simulink model "SoC"  (R2023b)
settings: Solver=FixedStepAuto  StartTime=0.0  StopTime=14000  RelTol=1e-3
libraries: BatteryEstimators x4
settings Model: Creator=dwegg  LastModifiedBy=joser
settings SolverCC: AlgebraicLoopSolver=TrustRegion
settings OptimizationCC: DefaultParameterBehavior=Inlined
settings DebuggingCC: UnconnectedInputMsg=warning  UnconnectedOutputMsg=warning  UnconnectedLineMsg=warning  ArithmeticOperatorsInVariantConditions=warning
settings ModelReferenceCC: EnableRefExpFcnMdlSchedulingChecks=on
settings SFSimCC: CustomCodeUndefinedFunction=UseInterfaceOnly
settings RTWCC: Description=INTECRIO Real-Time Target  SystemTargetFile=irt.tlc  TemplateMakefile=irt_default_tmf
settings STFCustomTargetCC: UtilityFuncGeneration=Shared location  MatFileLogging=on  GRTInterface=on  SystemTargetFile=irt.tlc
settings GRTTargetCC: UtilityFuncGeneration=Shared location  ParMdlRefBuildCompliant=off  CompOptLevelCompliant=off  ConcurrentExecutionCompliant=off  CombineOutputUpdateFcns=off  CPPClassGenCompliant=off  GRTInterface=on  UseToolchainInfoCompliant=off  GenerateASAP2=on

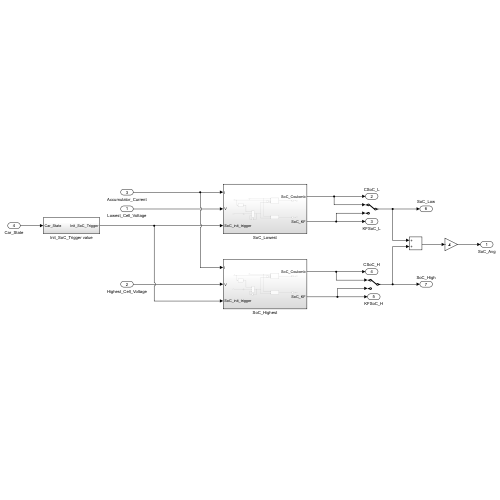
[thumbnail: Simulink's stored preview of the top-level diagram]
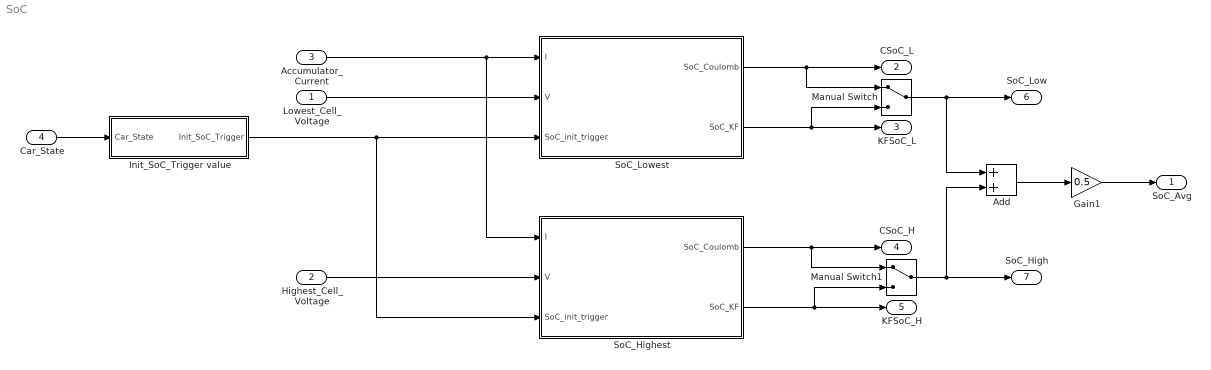
== system SoC ==
  Lowest_Cell_Voltage : Inport
  Highest_Cell_Voltage : Inport  Port=2
  Accumulator_Current : Inport  Port=3
  Car_State : Inport  Port=4
  Add : Sum
  Gain1 : Gain  Gain=0.5
  Init_SoC_Trigger value : Subsystem
  Manual Switch : ManualSwitch
  Manual Switch1 : ManualSwitch
  SoC_Highest : Subsystem
  SoC_Lowest : Subsystem
  SoC_Avg : Outport
  CSoC_L : Outport  Port=2
  KFSoC_L : Outport  Port=3
  CSoC_H : Outport  Port=4
  KFSoC_H : Outport  Port=5
  SoC_Low : Outport  Port=6
  SoC_High : Outport  Port=7
  wires:
  Lowest_Cell_Voltage/1 -> SoC_Lowest/2(V)
  Init_SoC_Trigger value/1(Init_SoC_Trigger) -> SoC_Highest/3(SoC_init_trigger), SoC_Lowest/3(SoC_init_trigger)
  Accumulator_Current/1 -> SoC_Highest/1(I), SoC_Lowest/1(I)
  SoC_Lowest/1(SoC_Coulomb) -> CSoC_L/1, Manual Switch/1
  SoC_Lowest/2(SoC_KF) -> KFSoC_L/1, Manual Switch/2
  SoC_Highest/2(SoC_KF) -> KFSoC_H/1, Manual Switch1/2
  SoC_Highest/1(SoC_Coulomb) -> CSoC_H/1, Manual Switch1/1
  Manual Switch/1 -> SoC_Low/1, Add/1
  Manual Switch1/1 -> SoC_High/1, Add/2
  Add/1 -> Gain1/1
  Gain1/1 -> SoC_Avg/1
  Highest_Cell_Voltage/1 -> SoC_Highest/2(V)
  Car_State/1 -> Init_SoC_Trigger value/1(Car_State)

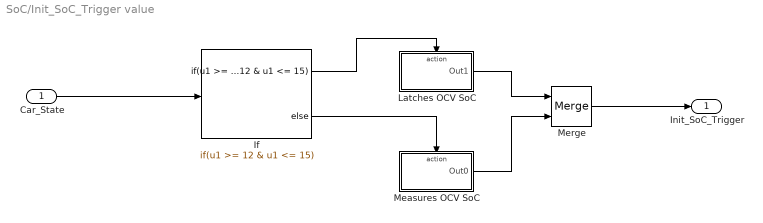
== system SoC/Init_SoC_Trigger value ==
  Car_State : Inport
  If : If  IfExpression=u1 >= 12 & u1 <= 15
  Latches OCV SoC : Subsystem  TreatAsAtomicUnit=on
  Measures OCV SoC : Subsystem  TreatAsAtomicUnit=on
  Merge : Merge
  Init_SoC_Trigger : Outport  VectorParamsAs1DForOutWhenUnconnected=off
  wires:
  Car_State/1 -> If/1
  If/1 -> Latches OCV SoC/Action
  If/2 -> Measures OCV SoC/Action
  Measures OCV SoC/1(Out0) -> Merge/2
  Latches OCV SoC/1(Out1) -> Merge/1
  Merge/1 -> Init_SoC_Trigger/1

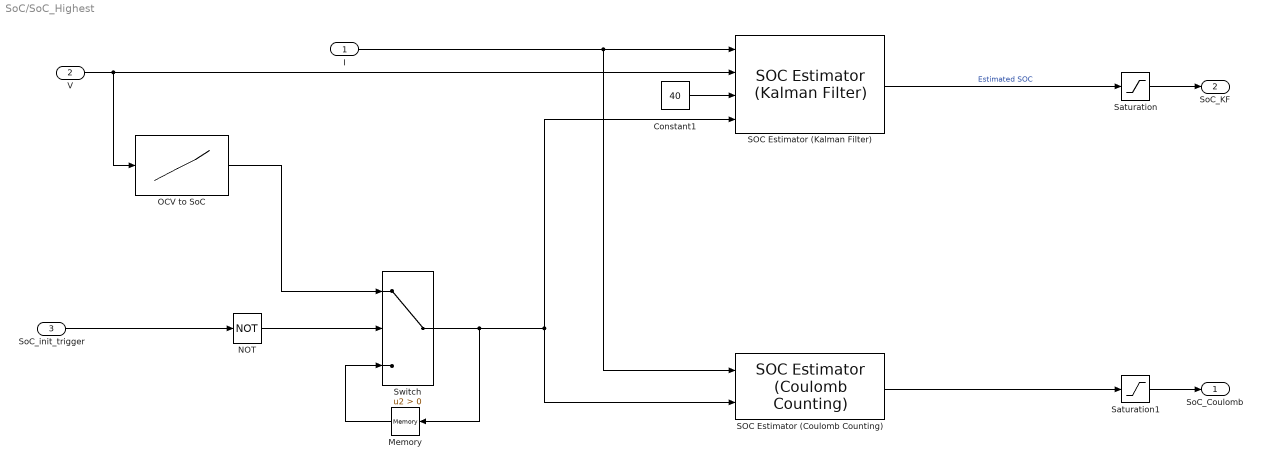
== system SoC/SoC_Highest ==
  I : Inport
  V : Inport  Port=2
  SoC_init_trigger : Inport  Port=3
  Constant1 : Constant  Value=40
  Memory : Memory
  NOT : Logic  Operator=NOT  IconShape=distinctive  AllPortsSameDT=off  OutDataTypeStr=boolean
  OCV to SoC : Lookup_n-D  NumberOfTableDimensions=1  BreakpointsForDimension1=|  Table=|  InternalRulePriority=Speed  RndMeth=Simplest
      BreakpointsForDimension1=|
      | [2.94959022892031
      | 3.21416977318498
      | 3.34338141328538
      | 3.38823547157865
      | 3.42107134634789
      | 3.48650481123582
      | 3.51335866761468
      | 3.54070339538832
      | 3.56968305677313
      | 3.63185877907628
      | 3.63255716896237
      | 3.64803371545993
      | 3.66548496788278
      | 3.66563518858557
      | 3.72681148156897
      | 3.76406010705888
      | 3.77075982343748
      | 3.84270466053206
      | 3.84295206305238
      | 3.90164564850831
      | 3.96498508551296
      | 3.96615700649565
      | 4.04797311953080
      | 4.07602027520885
      | 4.10936207844059
      | 4.18278376875771]
      Table=|
      | [0.00364887820512694
      | 0.0406322115384605
      | 0.0806891025641018
      | 0.120744391025641
      | 0.160802083333333
      | 0.200854967948718
      | 0.240911057692307
      | 0.280964743589743
      | 0.321025641025641
      | 0.361079326923077
      | 0.401137019230769
      | 0.441193910256410
      | 0.481247596153846
      | 0.521301282051282
      | 0.561357371794872
      | 0.601413461538462
      | 0.641456730769231
      | 0.681509615384616
      | 0.721566506410257
      | 0.761620993589744
      | 0.801677884615385
      | 0.841734775641026
      | 0.881788461538462
      | 0.921837339743590
      | 0.961899038461539
      | 0.998685256410256]
  SOC Estimator (Coulomb Counting) : BatteryEstimators/SOC Estimator (Coulomb Counting)  CurrentInputPartition=on  AH=2.6*5  Ts=1
  SOC Estimator (Kalman Filter) : BatteryEstimators/SOC Estimator (Kalman Filter)  CurrentInputPartition=off  filterType=Unscented Kalman filter  alpha=1  beta=2  kappa=0  Q=|  R=1e-3  P0=[1e-8 0; 0 1]  Ts=.025  SOC_vec=|  T_vec=[40+273]  R0_mat=|  R1_mat=|  tau1_mat=|  V0_mat=|  AH=12.5
      Q=|
      | [1e-9 0;
      | 0 1e-9]
      SOC_vec=|
      | [0.00364887820512694
      | 0.0406322115384605
      | 0.0806891025641018
      | 0.120744391025641
      | 0.160802083333333
      | 0.200854967948718
      | 0.240911057692307
      | 0.280964743589743
      | 0.321025641025641
      | 0.361079326923077
      | 0.401137019230769
      | 0.441193910256410
      | 0.481247596153846
      | 0.521301282051282
      | 0.561357371794872
      | 0.601413461538462
      | 0.641456730769231
      | 0.681509615384616
      | 0.721566506410257
      | 0.761620993589744
      | 0.801677884615385
      | 0.841734775641026
      | 0.881788461538462
      | 0.921837339743590
      | 0.961899038461539
      | 0.998685256410256]
      R0_mat=|
      | [0.0100233572019649
      | 0.0262776800968641
      | 0.0363128958641671
      | 0.0100113094505490
      | 0.0286486807277356
      | 0.0149767890889632
      | 0.0144578183036739
      | 0.0281525249750630
      | 0.0100063258437773
      | 0.0279749794813750
      | 0.0217631517067980
      | 0.0101315932150831
      | 0.0204969050806245
      | 0.0100036904397663
      | 0.0234196819492359
      | 0.0285785961250009
      | 0.0100010777636376
      | 0.0285512087508609
      | 0.0138948165245514
      | 0.0152455499563035
      | 0.0271834062533151
      | 0.00999543636151631
      | 0.0233190816650244
      | 0.0174459063712128
      | 0.00997795030699019
      | 0.0103822437854372]
      R1_mat=|
      | [0.000499569519126077
      | 0.000566384348175598
      | 0.000620513515330880
      | 0.000501834816986178
      | 0.000588952675343360
      | 0.000529656285954493
      | 0.000517421423028936
      | 0.000587687483006353
      | 0.000500912051109555
      | 0.000578364620913254
      | 0.000558041081149625
      | 0.000501034112890869
      | 0.000552539389402844
      | 0.000501551598015617
      | 0.000557375879673445
      | 0.000589089399714461
      | 0.000500612734241474
      | 0.000591500744740345
      | 0.000524954003879735
      | 0.000521737226573142
      | 0.000584978563699472
      | 0.000501333485097591
      | 0.000556455598375632
      | 0.000536187820761028
      | 0.000499639620215416
      | 0.000507199196258293]
      tau1_mat=|
      | [9.99999965128907
      | 9.98553115975498
      | 9.98319684629733
      | 9.99994867285566
      | 9.97472406054001
      | 9.99688938669185
      | 9.99522470508715
      | 9.98942560461659
      | 9.99999050049701
      | 9.99099110217109
      | 9.99738841102412
      | 9.99884730510879
      | 9.99441213972015
      | 9.99999487663704
      | 9.99510659168373
      | 9.99771333296480
      | 9.99992313725565
      | 9.99397201956115
      | 10.0015797566463
      | 9.99642521143648
      | 9.99339019420605
      | 9.99998885830201
      | 9.98301776831365
      | 9.99305327108613
      | 9.99970822142190
      | 9.99116677405533]
      V0_mat=|
      | [2.94959022892031
      | 3.21416977318498
      | 3.34338141328538
      | 3.38823547157865
      | 3.50107134634789
      | 3.48650481123582
      | 3.51335866761468
      | 3.58070339538832
      | 3.56968305677313
      | 3.63985877907628
      | 3.63255716896237
      | 3.62803371545993
      | 3.67548496788278
      | 3.66563518858557
      | 3.72681148156897
      | 3.76466010705888
      | 3.76075982343748
      | 3.85370466053206
      | 3.84295206305238
      | 3.90164564850831
      | 3.96498508551296
      | 3.96615700649565
      | 4.04797311953080
      | 4.07602027520885
      | 4.10936207844059
      | 4.18278376875771]
      link override Kalman Filter/EKBF/Jacobian/2-D Lookup Table C1: NumberOfTableDimensions=1
      link override Kalman Filter/EKBF/Jacobian/2-D Lookup Table R0: NumberOfTableDimensions=1
      link override Kalman Filter/EKBF/Jacobian/2-D Lookup Table R1: NumberOfTableDimensions=1
      link override Kalman Filter/EKBF/Jacobian/2-D Lookup Table V0: NumberOfTableDimensions=1
      link override Kalman Filter/EKBF/Jacobian/2-D Lookup Table dV0: NumberOfTableDimensions=1
      link override Kalman Filter/EKF/Jacobian/2-D Lookup Table C1: NumberOfTableDimensions=1
      link override Kalman Filter/EKF/Jacobian/2-D Lookup Table R0: NumberOfTableDimensions=1
      link override Kalman Filter/EKF/Jacobian/2-D Lookup Table R1: NumberOfTableDimensions=1
      link override Kalman Filter/EKF/Jacobian/2-D Lookup Table V0: NumberOfTableDimensions=1
      link override Kalman Filter/EKF/Jacobian/2-D Lookup Table dV0: NumberOfTableDimensions=1
      link override Kalman Filter/UKBF/Prediction-correction/Measurement function/Measurement function/OCV Table: NumberOfTableDimensions=1
      link override Kalman Filter/UKBF/Prediction-correction/Measurement function/Measurement function/R0 Table: NumberOfTableDimensions=1
      link override Kalman Filter/UKBF/Prediction-correction/State function/State function/C1: NumberOfTableDimensions=1
      link override Kalman Filter/UKBF/Prediction-correction/State function/State function/R1: NumberOfTableDimensions=1
      link override Kalman Filter/UKF/Prediction/Measurement function/Measurement function/OCV Table: NumberOfTableDimensions=1
      link override Kalman Filter/UKF/Prediction/Measurement function/Measurement function/R0 Table: NumberOfTableDimensions=1
      link override Kalman Filter/UKF/Prediction/State function/State function/C1: NumberOfTableDimensions=1
      link override Kalman Filter/UKF/Prediction/State function/State function/R1: NumberOfTableDimensions=1
  Saturation : Saturate  UpperLimit=100  LowerLimit=0
  Saturation1 : Saturate  UpperLimit=100  LowerLimit=0
  Switch : Switch  Criteria=u2 > Threshold  ZeroCross=off  SaturateOnIntegerOverflow=off  InputSameDT=off
  SoC_Coulomb : Outport  VectorParamsAs1DForOutWhenUnconnected=off
  SoC_KF : Outport  Port=2
  wires:
  Saturation1/1 -> SoC_Coulomb/1
  Saturation/1 -> SoC_KF/1
  SoC_init_trigger/1 -> NOT/1
  NOT/1 -> Switch/2
  Memory/1 -> Switch/3
  OCV to SoC/1 -> Switch/1
  V/1 -> SOC Estimator (Kalman Filter)/2, OCV to SoC/1
  Switch/1 -> SOC Estimator (Coulomb Counting)/2, SOC Estimator (Kalman Filter)/4, Memory/1
  I/1 -> SOC Estimator (Kalman Filter)/1, SOC Estimator (Coulomb Counting)/1
  Constant1/1 -> SOC Estimator (Kalman Filter)/3
  SOC Estimator (Kalman Filter)/1 -> Saturation/1  "Estimated SOC"
  SOC Estimator (Coulomb Counting)/1 -> Saturation1/1

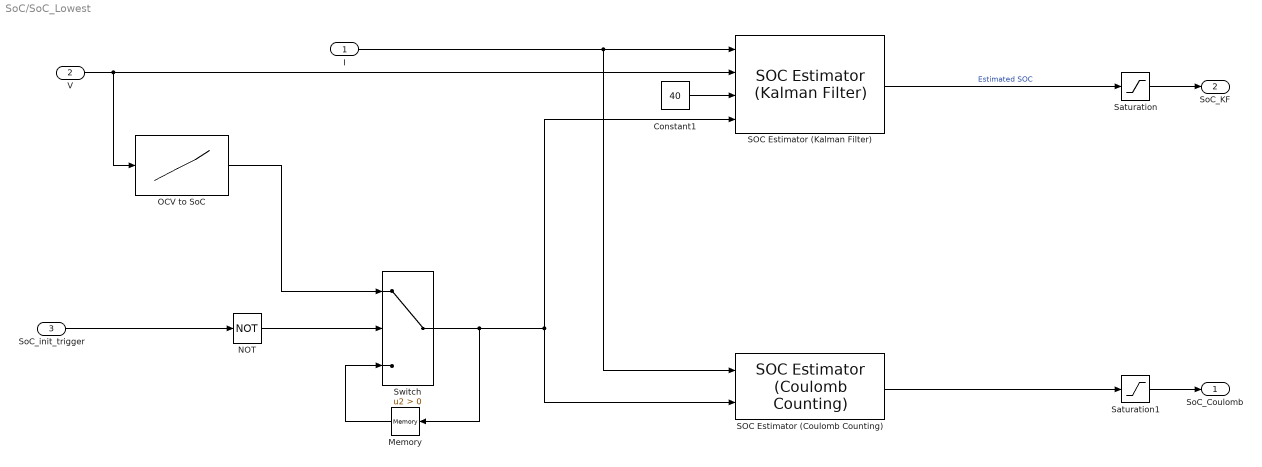
== system SoC/SoC_Lowest ==
  I : Inport
  V : Inport  Port=2
  SoC_init_trigger : Inport  Port=3
  Constant1 : Constant  Value=40
  Memory : Memory
  NOT : Logic  Operator=NOT  IconShape=distinctive  AllPortsSameDT=off  OutDataTypeStr=boolean
  OCV to SoC : Lookup_n-D  NumberOfTableDimensions=1  BreakpointsForDimension1=|  Table=|  InternalRulePriority=Speed  RndMeth=Simplest
      BreakpointsForDimension1=|
      | [2.94959022892031
      | 3.21416977318498
      | 3.34338141328538
      | 3.38823547157865
      | 3.42107134634789
      | 3.48650481123582
      | 3.51335866761468
      | 3.54070339538832
      | 3.56968305677313
      | 3.63185877907628
      | 3.63255716896237
      | 3.64803371545993
      | 3.66548496788278
      | 3.66563518858557
      | 3.72681148156897
      | 3.76406010705888
      | 3.77075982343748
      | 3.84270466053206
      | 3.84295206305238
      | 3.90164564850831
      | 3.96498508551296
      | 3.96615700649565
      | 4.04797311953080
      | 4.07602027520885
      | 4.10936207844059
      | 4.18278376875771]
      Table=|
      | [0.00364887820512694
      | 0.0406322115384605
      | 0.0806891025641018
      | 0.120744391025641
      | 0.160802083333333
      | 0.200854967948718
      | 0.240911057692307
      | 0.280964743589743
      | 0.321025641025641
      | 0.361079326923077
      | 0.401137019230769
      | 0.441193910256410
      | 0.481247596153846
      | 0.521301282051282
      | 0.561357371794872
      | 0.601413461538462
      | 0.641456730769231
      | 0.681509615384616
      | 0.721566506410257
      | 0.761620993589744
      | 0.801677884615385
      | 0.841734775641026
      | 0.881788461538462
      | 0.921837339743590
      | 0.961899038461539
      | 0.998685256410256]
  SOC Estimator (Coulomb Counting) : BatteryEstimators/SOC Estimator (Coulomb Counting)  CurrentInputPartition=on  AH=2.6*5  Ts=1
  SOC Estimator (Kalman Filter) : BatteryEstimators/SOC Estimator (Kalman Filter)  CurrentInputPartition=off  filterType=Extended Kalman filter  alpha=1  beta=2  kappa=0  Q=|  R=1e-3  P0=[1e-8 0; 0 1]  Ts=.025  SOC_vec=|  T_vec=[40+273]  R0_mat=|  R1_mat=|  tau1_mat=|  V0_mat=|  AH=12.5
      Q=|
      | [1e-9 0;
      | 0 1e-9]
      SOC_vec=|
      | [0.00364887820512694
      | 0.0406322115384605
      | 0.0806891025641018
      | 0.120744391025641
      | 0.160802083333333
      | 0.200854967948718
      | 0.240911057692307
      | 0.280964743589743
      | 0.321025641025641
      | 0.361079326923077
      | 0.401137019230769
      | 0.441193910256410
      | 0.481247596153846
      | 0.521301282051282
      | 0.561357371794872
      | 0.601413461538462
      | 0.641456730769231
      | 0.681509615384616
      | 0.721566506410257
      | 0.761620993589744
      | 0.801677884615385
      | 0.841734775641026
      | 0.881788461538462
      | 0.921837339743590
      | 0.961899038461539
      | 0.998685256410256]
      R0_mat=|
      | [0.0100233572019649
      | 0.0262776800968641
      | 0.0363128958641671
      | 0.0100113094505490
      | 0.0286486807277356
      | 0.0149767890889632
      | 0.0144578183036739
      | 0.0281525249750630
      | 0.0100063258437773
      | 0.0279749794813750
      | 0.0217631517067980
      | 0.0101315932150831
      | 0.0204969050806245
      | 0.0100036904397663
      | 0.0234196819492359
      | 0.0285785961250009
      | 0.0100010777636376
      | 0.0285512087508609
      | 0.0138948165245514
      | 0.0152455499563035
      | 0.0271834062533151
      | 0.00999543636151631
      | 0.0233190816650244
      | 0.0174459063712128
      | 0.00997795030699019
      | 0.0103822437854372]
      R1_mat=|
      | [0.000499569519126077
      | 0.000566384348175598
      | 0.000620513515330880
      | 0.000501834816986178
      | 0.000588952675343360
      | 0.000529656285954493
      | 0.000517421423028936
      | 0.000587687483006353
      | 0.000500912051109555
      | 0.000578364620913254
      | 0.000558041081149625
      | 0.000501034112890869
      | 0.000552539389402844
      | 0.000501551598015617
      | 0.000557375879673445
      | 0.000589089399714461
      | 0.000500612734241474
      | 0.000591500744740345
      | 0.000524954003879735
      | 0.000521737226573142
      | 0.000584978563699472
      | 0.000501333485097591
      | 0.000556455598375632
      | 0.000536187820761028
      | 0.000499639620215416
      | 0.000507199196258293]
      tau1_mat=|
      | [9.99999965128907
      | 9.98553115975498
      | 9.98319684629733
      | 9.99994867285566
      | 9.97472406054001
      | 9.99688938669185
      | 9.99522470508715
      | 9.98942560461659
      | 9.99999050049701
      | 9.99099110217109
      | 9.99738841102412
      | 9.99884730510879
      | 9.99441213972015
      | 9.99999487663704
      | 9.99510659168373
      | 9.99771333296480
      | 9.99992313725565
      | 9.99397201956115
      | 10.0015797566463
      | 9.99642521143648
      | 9.99339019420605
      | 9.99998885830201
      | 9.98301776831365
      | 9.99305327108613
      | 9.99970822142190
      | 9.99116677405533]
      V0_mat=|
      | [2.94959022892031
      | 3.21416977318498
      | 3.34338141328538
      | 3.38823547157865
      | 3.50107134634789
      | 3.48650481123582
      | 3.51335866761468
      | 3.58070339538832
      | 3.56968305677313
      | 3.63985877907628
      | 3.63255716896237
      | 3.62803371545993
      | 3.67548496788278
      | 3.66563518858557
      | 3.72681148156897
      | 3.76466010705888
      | 3.76075982343748
      | 3.85370466053206
      | 3.84295206305238
      | 3.90164564850831
      | 3.96498508551296
      | 3.96615700649565
      | 4.04797311953080
      | 4.07602027520885
      | 4.10936207844059
      | 4.18278376875771]
      link override Kalman Filter/EKBF/Jacobian/2-D Lookup Table C1: NumberOfTableDimensions=1
      link override Kalman Filter/EKBF/Jacobian/2-D Lookup Table R0: NumberOfTableDimensions=1
      link override Kalman Filter/EKBF/Jacobian/2-D Lookup Table R1: NumberOfTableDimensions=1
      link override Kalman Filter/EKBF/Jacobian/2-D Lookup Table V0: NumberOfTableDimensions=1
      link override Kalman Filter/EKBF/Jacobian/2-D Lookup Table dV0: NumberOfTableDimensions=1
      link override Kalman Filter/EKF/Jacobian/2-D Lookup Table C1: NumberOfTableDimensions=1
      link override Kalman Filter/EKF/Jacobian/2-D Lookup Table R0: NumberOfTableDimensions=1
      link override Kalman Filter/EKF/Jacobian/2-D Lookup Table R1: NumberOfTableDimensions=1
      link override Kalman Filter/EKF/Jacobian/2-D Lookup Table V0: NumberOfTableDimensions=1
      link override Kalman Filter/EKF/Jacobian/2-D Lookup Table dV0: NumberOfTableDimensions=1
      link override Kalman Filter/UKBF/Prediction-correction/Measurement function/Measurement function/OCV Table: NumberOfTableDimensions=1
      link override Kalman Filter/UKBF/Prediction-correction/Measurement function/Measurement function/R0 Table: NumberOfTableDimensions=1
      link override Kalman Filter/UKBF/Prediction-correction/State function/State function/C1: NumberOfTableDimensions=1
      link override Kalman Filter/UKBF/Prediction-correction/State function/State function/R1: NumberOfTableDimensions=1
      link override Kalman Filter/UKF/Prediction/Measurement function/Measurement function/OCV Table: NumberOfTableDimensions=1
      link override Kalman Filter/UKF/Prediction/Measurement function/Measurement function/R0 Table: NumberOfTableDimensions=1
      link override Kalman Filter/UKF/Prediction/State function/State function/C1: NumberOfTableDimensions=1
      link override Kalman Filter/UKF/Prediction/State function/State function/R1: NumberOfTableDimensions=1
  Saturation : Saturate  UpperLimit=100  LowerLimit=0
  Saturation1 : Saturate  UpperLimit=100  LowerLimit=0
  Switch : Switch  Criteria=u2 > Threshold  ZeroCross=off  SaturateOnIntegerOverflow=off  InputSameDT=off
  SoC_Coulomb : Outport  VectorParamsAs1DForOutWhenUnconnected=off
  SoC_KF : Outport  Port=2
  wires:
  SOC Estimator (Coulomb Counting)/1 -> Saturation1/1
  SOC Estimator (Kalman Filter)/1 -> Saturation/1  "Estimated SOC"
  Constant1/1 -> SOC Estimator (Kalman Filter)/3
  I/1 -> SOC Estimator (Coulomb Counting)/1, SOC Estimator (Kalman Filter)/1
  Switch/1 -> Memory/1, SOC Estimator (Kalman Filter)/4, SOC Estimator (Coulomb Counting)/2
  V/1 -> OCV to SoC/1, SOC Estimator (Kalman Filter)/2
  OCV to SoC/1 -> Switch/1
  Memory/1 -> Switch/3
  NOT/1 -> Switch/2
  SoC_init_trigger/1 -> NOT/1
  Saturation/1 -> SoC_KF/1
  Saturation1/1 -> SoC_Coulomb/1

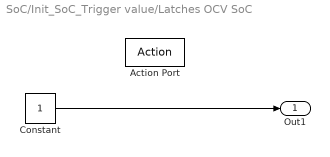
== system SoC/Init_SoC_Trigger value/Latches OCV SoC ==
  Action Port : ActionPort  ActionPortLabel=if(u1 >= 12 & u1 <= 15)
  Constant : Constant
  Out1 : Outport  VectorParamsAs1DForOutWhenUnconnected=off
  wires:
  Constant/1 -> Out1/1

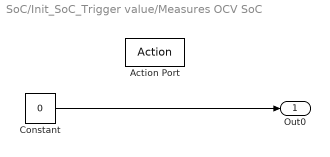
== system SoC/Init_SoC_Trigger value/Measures OCV SoC ==
  Action Port : ActionPort  ActionPortLabel=else
  Constant : Constant  Value=0
  Out0 : Outport  VectorParamsAs1DForOutWhenUnconnected=off
  wires:
  Constant/1 -> Out0/1
